simulink model "model04"  (R2018b)
settings: Solver=ode4  StartTime=0.0  StopTime=5  FixedStep=0.001  RelTol=1e-3
values from neighbouring files (symbols this model uses):
  k1 = b^2/((V^2*sin(lambda)-b*g*cos(lambda))*m*a*c*sin(lambda))    [main.m]    (also in plotRlocus.m = 0.06)
  k2 = b*g/(V^2*sin(lambda)-b*g*cos(lambda))    [main.m]    (also in plotRlocus.m = 1.95)
undefined symbols (not defined in the file or in its folder): denG_delta_T, denG_eta_T, denG_psi_delta, denK, numG_delta_T, numG_eta_T, numG_psi_delta, numK
settings Model: Creator=franc  LastModifiedBy=franc

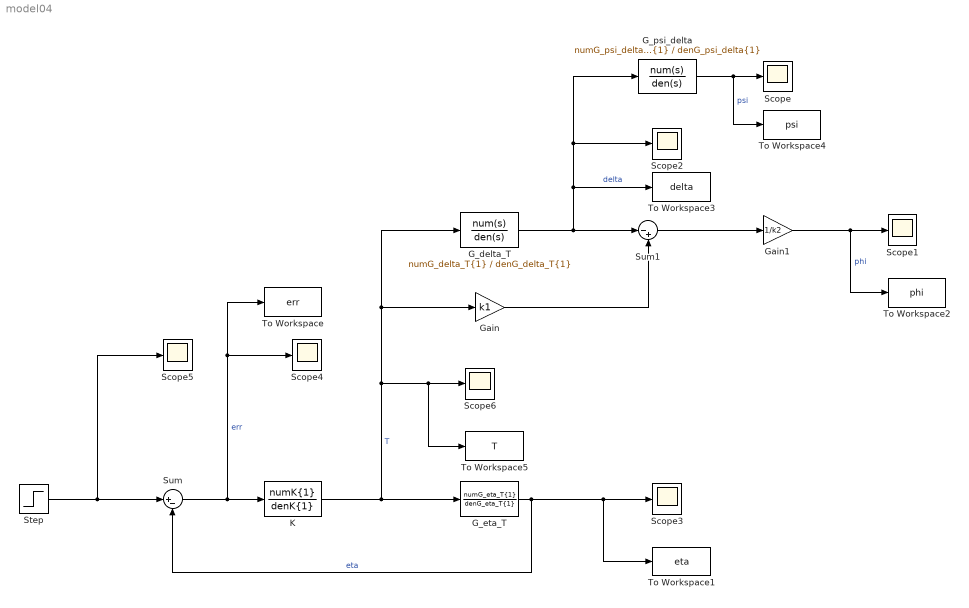
== system model04 ==
  G_delta_T : TransferFcn  Numerator=numG_delta_T{1}  Denominator=denG_delta_T{1}
  G_eta_T : TransferFcn  Numerator=numG_eta_T{1}  Denominator=denG_eta_T{1}
  G_psi_delta : TransferFcn  Numerator=numG_psi_delta{1}  Denominator=denG_psi_delta{1}
  Gain : Gain  Gain=k1
  Gain1 : Gain  Gain=1/k2
  K : TransferFcn  Numerator=numK{1}  Denominator=denK{1}
  Scope{,1..6} (7 alike) : Scope
  Step : Step  Time=0  After=2  SampleTime=0
  Sum : Sum  Inputs=|+-
  Sum1 : Sum  Inputs=|-+
  To Workspace : ToWorkspace  VariableName=err  SaveFormat=Timeseries  SampleTime=-1
  To Workspace1 : ToWorkspace  VariableName=eta  SaveFormat=Timeseries  SampleTime=-1
  To Workspace2 : ToWorkspace  VariableName=phi  SaveFormat=Timeseries  SampleTime=-1
  To Workspace3 : ToWorkspace  VariableName=delta  SaveFormat=Timeseries  SampleTime=-1
  To Workspace4 : ToWorkspace  VariableName=psi  SaveFormat=Timeseries  SampleTime=-1
  To Workspace5 : ToWorkspace  VariableName=T  SaveFormat=Timeseries  SampleTime=-1
  wires:
  Sum1/1 -> Gain1/1
  G_delta_T/1 -> To Workspace3/1, Scope2/1, G_psi_delta/1, Sum1/1  "delta"
  Gain/1 -> Sum1/2
  G_psi_delta/1 -> To Workspace4/1, Scope/1  "psi"
  Gain1/1 -> To Workspace2/1, Scope1/1  "phi"
  G_eta_T/1 -> To Workspace1/1, Scope3/1, Sum/2  "eta"
  Sum/1 -> To Workspace/1, Scope4/1, K/1  "err"
  Step/1 -> Scope5/1, Sum/1
  K/1 -> Scope6/1, To Workspace5/1, Gain/1, G_delta_T/1, G_eta_T/1  "T"
